simulink library "EMPSMD3E01MSEREF"  (R2014b)
settings: Solver=ode45  StartTime=0.0  StopTime=10.0  RelTol=1e-3
settings Model: Creator=vda2sh  LastModifiedBy=vda2sh

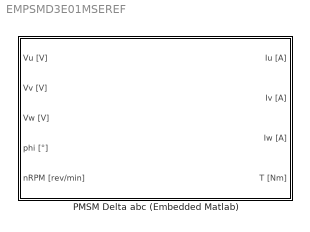
== system EMPSMD3E01MSEREF ==
  PMSM Delta abc (Embedded Matlab) : Subsystem  Tag=EMPSMD3E01MSEREF  mask(EMPSMD3E01MSEREF){N=2, r_m=0.1, l=[1e-4 0 0.1e-4 0 0], m=[1e-5 0 0.1e-5 0 0], Km=0.005, a357=[1/9 1/25 1/49]*5e-3, xIainit=0.0, xIbinit=0.0, xIcinit=0.0}
      mask prompts: N "Number of pole pairs   N"; r_m "Winding resistance   R [Ohm]"; l "Self inductance   [l0 l1 l2 l3...] [H]"; m "Mutal inductance   [m0 m1 m2 m3...] [H]"; Km "Fundamental of flux   Km [Vs]"; a357 "Flux harmonic  [a3 a5 a7...] [Vs]"; xIainit "Initial Stator current, phase a [A]"; xIbinit "Initial Stator current, phase b [A]"; xIcinit "Initial Stator current, phase c [A]"
      mask help:
      | EMPSMD3E01MSEREF - PMSM Delta abc (Embedded Matlab)
      |
      | This is a model of a permanent magnetic synchronous machine in abc-coordinates in delta connection with linear magnetic conditions.
      settings: AttributesFormatString=<%<Tag>>
      mask Help: eval('show_docs_mseref_emachines(''EMPSMD3E01MSEREF'')')
      mask Display:
      | image(imread('EMPSMD301MSEREF.png'),[0.25,0.2,0.5,0.7])
      | text(0.6,0.1, 'MSE')
      | port_label('input',1,'Vu [V]')
      | port_label('input',2,'Vv [V]')
      | port_label('input',3,'Vw [V]')
      | port_label('input',4,'phi [°]')
      | port_label('input',5,'nRPM [rev/min]')
      | port_label('output',1,'Iu [A]')
      | port_label('output',2,'Iv [A]')
      | port_label('output',3,'Iw [A]')
      | port_label('output',4,'T [Nm]')

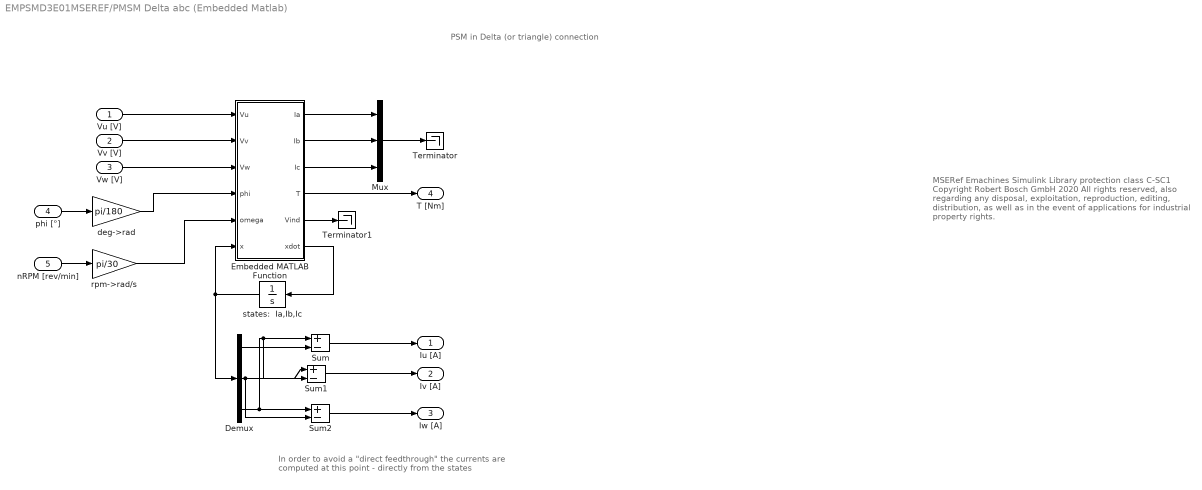
== system EMPSMD3E01MSEREF/PMSM Delta abc (Embedded Matlab) ==
  note: In order to avoid a "direct feedthrough" the currents
      | are computed at this point - directly from the states
  note: PSM in Delta (or triangle) connection
  note: MSERef Emachines Simulink Library
      | protection class C-SC1
      |
      | Copyright Robert Bosch GmbH 2020
      |
      | All rights reserved, also regarding any disposal, exploitation,
      | reproduction, editing, distribution, as well as in the event of
      | applications for industrial property rights.
  Vu [V] : Inport
  Vv [V] : Inport  Port=2
  Vw [V] : Inport  Port=3
  phi [°] : Inport  Port=4
  nRPM [rev/min] : Inport  Port=5
  Demux : Demux  Outputs=3
  Embedded MATLAB Function : MATLAB Function  TreatAsAtomicUnit=on
  Mux : Mux  Inputs=3
  Sum : Sum  Inputs=+-
  Sum1 : Sum  Inputs=+-
  Sum2 : Sum  Inputs=+-
  Terminator : Terminator
  Terminator1 : Terminator
  deg->rad : Gain  Gain=pi/180
  rpm->rad/s : Gain  Gain=pi/30
  states:  Ia,Ib,Ic : Integrator  InitialCondition=[xIainit xIbinit xIcinit]
  Iu [A] : Outport
  Iv [A] : Outport  Port=2
  Iw [A] : Outport  Port=3
  T [Nm] : Outport  Port=4
  wires:
  Embedded MATLAB Function/3(Ic) -> Mux/3
  Embedded MATLAB Function/2(Ib) -> Mux/2
  Embedded MATLAB Function/1(Ia) -> Mux/1
  rpm->rad/s/1 -> Embedded MATLAB Function/5(omega)
  deg->rad/1 -> Embedded MATLAB Function/4(phi)
  Embedded MATLAB Function/6(xdot) -> states:  Ia,Ib,Ic/1
  states:  Ia,Ib,Ic/1 -> Embedded MATLAB Function/6(x), Demux/1
  Vu [V]/1 -> Embedded MATLAB Function/1(Vu)
  Vv [V]/1 -> Embedded MATLAB Function/2(Vv)
  Vw [V]/1 -> Embedded MATLAB Function/3(Vw)
  phi [°]/1 -> deg->rad/1
  nRPM [rev/min]/1 -> rpm->rad/s/1
  Embedded MATLAB Function/4(T) -> T [Nm]/1
  Demux/1 -> Sum/1, Sum1/2
  Demux/3 -> Sum/2, Sum2/1
  Sum/1 -> Iu [A]/1
  Sum1/1 -> Iv [A]/1
  Demux/2 -> Sum1/1, Sum2/2
  Sum2/1 -> Iw [A]/1
  Mux/1 -> Terminator/1
  Embedded MATLAB Function/5(Vind) -> Terminator1/1

== matlab function EMPSMD3E01MSEREF/PMSM Delta abc (Embedded Matlab)/Embedded MATLAB Function ==
  data: Vu input; Vv input; Vw input; phi input; omega input; Ia output; Ib output; Ic output; T output; Vind output; Km parameter; a357 parameter; N parameter; l parameter; m parameter; r_m parameter; x input; xdot output
function [Ia, Ib, Ic, T,Vind,xdot ] = fcn(Vu,Vv,Vw, phi, omega, Km, a357,N, l, m,r_m, x)

% MSE Reference Model Library
% 
% This template is created by:                                                 
% ROBERT BOSCH GmbH, Stuttgart, Germany, Dept. CR/AEH3
%                                                                              
% Robert Bosch Proprietary 
% 
% All rights reserved, also regarding any disposal, disclosure, exploitation , 
% reproduction, editing as well as in the event of applications for industrial 
% property rights.                                                                        
% This template may not be reproduced in any way (physically or electronically)
% without prior written permission from Robert Bosch GmbH. The content of this 
% template is subject to change without notice.                                
% Robert Bosch GmbH does not assume liability for the use of this template or  
% the results obtained from using it.                                          

%% States are x=[Ia, Ib, Ic]
Ia=x(1); 
Ib=x(2);
Ic=x(3);

%% Angle dependance of parameters %%
N_l=length(l);
N_m=length(m);
N_a357=length(a357);
%Angle dependance of the inductance 
k1=[0:N_l-1];
k2=[0:N_m-1];
la  = sum(cos(k1*N*phi).*l);                %la=l(1)+l(2)*cos(phi*N)+l(3)*cos(2*phi*N)+...
lb  = sum(cos(k1*N*(phi-2*pi/3/N)).*l);     %Equation (6)
lc  = sum(cos(k1*N*(phi+2*pi/3/N)).*l);
mbc = sum(cos(k2*N*phi).*m);                %Equation (7)
mac = sum(cos(k2*N*(phi-2*pi/3/N)).*m);
mab = sum(cos(k2*N*(phi+2*pi/3/N)).*m);
%derivative of the inductance w.r.t phi
dla  = sum(N*k1.*-sin(k1*N*phi).*l);
dlb  = sum(N*k1.*-sin(k1*N*(phi-2*pi/3/N)).*l);
dlc  = sum(N*k1.*-sin(k1*N*(phi+2*pi/3/N)).*l);
dmbc = sum(N*k2.*-sin(k2*N*phi).*m);
dmac = sum(N*k2.*-sin(k2*N*(phi-2*pi/3/N)).*m);
dmab = sum(N*k2.*-sin(k2*N*(phi+2*pi/3/N)).*m);
%derivative of the flux w.r.t phi
k3=2*[0:N_a357]+1;
dPsia_pm = sum(N*k3.*-sin(k3*N*phi).*[Km a357]);            %derivative of equation (9)
dPsib_pm = sum(N*k3.*-sin(k3.*N*(phi-2*pi/3/N)).*[Km a357]);
dPsic_pm = sum(N*k3.*-sin(k3.*N*(phi+2*pi/3/N)).*[Km a357]);
%% Definition of matrices+vectors %%
L  = [la -mab -mac; -mab lb -mbc;-mac -mbc lc];             %Equation (5)
Linv=inv(L);
dL = [dla -dmab -dmac; -dmab dlb -dmbc;-dmac -dmbc dlc];
dPSI_pm  =[dPsia_pm; dPsib_pm; dPsic_pm];
I  = [Ia;Ib;Ic];
R=r_m*eye(3);
Vdiff=[Vu-Vv;Vv-Vw;Vw-Vu];
%% Torque %%
T=dPSI_pm'*I+1/2*I'*dL*I;                       %Equation (4)
%% Inducted voltage%%
Vind=(dPSI_pm+dL*I)*omega;
%% Derivative of the states (currents) %%
xdot=Linv*(Vdiff-R*I-Vind);                     %Equation (1)
